simulink model "BrowarModel"  (R2024a)
settings: Solver=ode5  StartTime=0.0  StopTime=inf  FixedStep=0.1  RelTol=1e-3
undefined symbols (not defined in the file or in its folder): localhost, Matrikon, OI
libraries: opclib x24
(part 1 of 9)
settings Model: Creator=Administrator  LastModifiedBy=user
settings SolverCC: AlgebraicLoopSolver=TrustRegion
settings DataIOCC: LimitDataPoints=on  SaveFormat=Array  SignalLoggingSaveFormat=ModelDataLogs  ReturnWorkspaceOutputs=off
settings OptimizationCC: BlockReduction=off  BooleanDataType=off  BufferReuse=off  ExpressionDepthLimit=2147483647  InitFltsAndDblsToZero=on  LifeSpan=inf
settings DebuggingCC: UnderspecifiedInitializationDetection=Classic  MergeDetectMultiDrivingBlocksExec=none  SolverPrmCheckMsg=warning  FcnCallInpInsideContextMsg=warning  UnconnectedInputMsg=warning  UnconnectedOutputMsg=warning  UnconnectedLineMsg=warning  StateNameClashWarn=warning  SFUnexpectedBacktrackingDiag=warning  SFNoUnconditionalDefaultTransitionDiag=warning  SFExecutionAtInitializationDiag=none  ArithmeticOperatorsInVariantConditions=warning
settings HardwareCC: ProdBitPerPointer=32  ProdBitPerSizeT=32  ProdBitPerPtrDiffT=32  ProdLargestAtomicFloat=None  ProdIntDivRoundTo=Undefined  ProdEndianess=Unspecified  ProdWordSize=32  ProdHWDeviceType=32-bit Generic
settings ModelReferenceCC: EnableRefExpFcnMdlSchedulingChecks=on  PropagateSignalLabelsOutOfModel=off
settings SFSimCC: SimUseLocalCustomCode=off  CustomCodeUndefinedFunction=UseInterfaceOnly
settings RTWCC: RTWUseLocalCustomCode=off  GPUComputeCapability=3.5  DLArmComputeVersion=19.05
settings CodeAppCC: StateflowObjectComments=on
settings GRTTargetCC: TargetLangStandard=C89/C90 (ANSI)  CombineOutputUpdateFcns=off  GRTInterface=on
settings ConfigComp: CovMetricSettings=dw  CovSaveCumulativeToWorkspaceVar=on  CovSaveSingleToWorkspaceVar=on  CovExternalEMLEnable=off

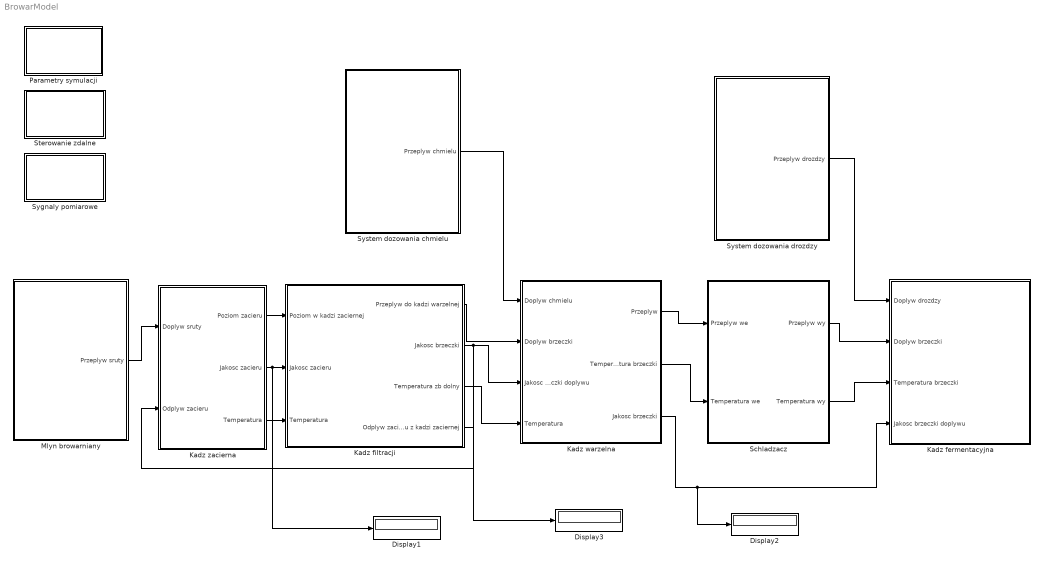
== system BrowarModel ==
  Display1 : Display
  Display2 : Display
  Display3 : Display
  Kadz fermentacyjna : Subsystem
  Kadz filtracji : Subsystem
  Kadz warzelna : Subsystem
  Kadz zacierna : Subsystem
  Mlyn browarniany : Subsystem
  Parametry symulacji : Subsystem
  Schladzacz : Subsystem
  Sterowanie zdalne : Subsystem
  Sygnaly pomiarowe : Subsystem
  System dozowania chmielu : Subsystem
  System dozowania drozdzy : Subsystem
  wires:
  Kadz filtracji/1(Przeplyw do kadzi warzelnej) -> Kadz warzelna/2(Doplyw brzeczki)
  System dozowania chmielu/1(Przeplyw chmielu) -> Kadz warzelna/1(Doplyw chmielu)
  Kadz warzelna/3(Jakosc brzeczki) -> Kadz fermentacyjna/4(Jakosc brzeczki doplywu), Display2/1
  Kadz filtracji/3(Temperatura zb dolny) -> Kadz warzelna/4(Temperatura)
  Kadz filtracji/2(Jakosc brzeczki) -> Kadz warzelna/3(Jakosc brzeczki doplywu), Display3/1
  Schladzacz/2(Temperatura wy) -> Kadz fermentacyjna/3(Temperatura brzeczki)
  Schladzacz/1(Przeplyw wy) -> Kadz fermentacyjna/2(Doplyw brzeczki)
  Kadz warzelna/1(Przeplyw) -> Schladzacz/1(Przeplyw we)
  Kadz warzelna/2(Temperatura brzeczki) -> Schladzacz/2(Temperatura we)
  System dozowania drozdzy/1(Przeplyw drozdzy) -> Kadz fermentacyjna/1(Doplyw drozdzy)
  Kadz filtracji/4(Odplyw zacieru z kadzi zaciernej) -> Kadz zacierna/2(Odplyw zacieru)
  Mlyn browarniany/1("Przeplyw sruty ") -> Kadz zacierna/1(Doplyw sruty)
  Kadz zacierna/1(Poziom zacieru) -> Kadz filtracji/1(Poziom w kadzi zaciernej)
  Kadz zacierna/2(Jakosc zacieru) -> Kadz filtracji/2(Jakosc zacieru), Display1/1
  Kadz zacierna/3(Temperatura) -> Kadz filtracji/3(Temperatura)

== system BrowarModel/Kadz fermentacyjna ==
  note: Kadz fermentacji
  Doplyw drozdzy : Inport
  Doplyw brzeczki : Inport  Port=2
  Temperatura brzeczki : Inport  Port=3
  Jakosc brzeczki doplywu : Inport  Port=4
  ET704 : Subsystem  mask{SrcZakres=12, Zakres=12, Kompensacja=0, ZakloceniaPom=off}
      mask prompts: SrcZakres "Zakres zmiennej w modelu"; Zakres "Zakres pomiarowy przetwornika pomiarowego"; Kompensacja "Kompensacja przetwornika pomiarowego"; ZakloceniaPom "Zaklocenia pomiarowe"
  ET705 : Subsystem  mask{SrcZakres=12, Zakres=12, Kompensacja=0, ZakloceniaPom=off}
      mask prompts: SrcZakres "Zakres zmiennej w modelu"; Zakres "Zakres pomiarowy przetwornika pomiarowego"; Kompensacja "Kompensacja przetwornika pomiarowego"; ZakloceniaPom "Zaklocenia pomiarowe"
  FV705 : Subsystem
  FV705SP : Subsystem
  FV706 : Subsystem
  Kadz fermentacyjna : Subsystem
  LT701 : Subsystem  mask{SrcZakres=3.5, Zakres=3.5, Kompensacja=0, ZakloceniaPom=on}
      mask prompts: SrcZakres "Zakres zmiennej w modelu"; Zakres "Zakres pomiarowy przetwornika pomiarowego"; Kompensacja "Kompensacja przetwornika pomiarowego"; ZakloceniaPom "Zaklocenia pomiarowe"
  LT701H : Subsystem
  LT701L : Subsystem
  ST704 : Subsystem  mask{SrcZakres=2000, Zakres=2000, Kompensacja=0, ZakloceniaPom=off}
      mask prompts: SrcZakres "Zakres zmiennej w modelu"; Zakres "Zakres pomiarowy przetwornika pomiarowego"; Kompensacja "Kompensacja przetwornika pomiarowego"; ZakloceniaPom "Zaklocenia pomiarowe"
  ST705 : Subsystem  mask{SrcZakres=2000, Zakres=2000, Kompensacja=0, ZakloceniaPom=off}
      mask prompts: SrcZakres "Zakres zmiennej w modelu"; Zakres "Zakres pomiarowy przetwornika pomiarowego"; Kompensacja "Kompensacja przetwornika pomiarowego"; ZakloceniaPom "Zaklocenia pomiarowe"
  TT702H : Subsystem  mask{SrcZakres=150, Zakres=150, Kompensacja=0, ZakloceniaPom=on}
      mask prompts: SrcZakres "Zakres zmiennej w modelu"; Zakres "Zakres pomiarowy przetwornika pomiarowego"; Kompensacja "Kompensacja przetwornika pomiarowego"; ZakloceniaPom "Zaklocenia pomiarowe"
  TT702L : Subsystem  mask{SrcZakres=150, Zakres=150, Kompensacja=0, ZakloceniaPom=on}
      mask prompts: SrcZakres "Zakres zmiennej w modelu"; Zakres "Zakres pomiarowy przetwornika pomiarowego"; Kompensacja "Kompensacja przetwornika pomiarowego"; ZakloceniaPom "Zaklocenia pomiarowe"
  TT702M : Subsystem  mask{SrcZakres=150, Zakres=150, Kompensacja=0, ZakloceniaPom=on}
      mask prompts: SrcZakres "Zakres zmiennej w modelu"; Zakres "Zakres pomiarowy przetwornika pomiarowego"; Kompensacja "Kompensacja przetwornika pomiarowego"; ZakloceniaPom "Zaklocenia pomiarowe"
  TV702 : Subsystem
  Terminator : Terminator
  XV704 : Subsystem
  XV704SP : Subsystem
  tag scope: ET704=global, ET705=global, LT701=global, LT701H=global, LT701L=global, Odplyw=global, ST704=global, ST705=global, TT702H=global, TT702L=global, TT702M=global, XV704Alarm=global, XV704Idle=global, XV704Running=global, XV705Alarm=global, XV705Idle=global, XV705Running=global
  wires:
  Kadz fermentacyjna/1(Poziom) -> LT701/1(In)
  Kadz fermentacyjna/2(Poziom wysoki) -> LT701H/1(In)
  Kadz fermentacyjna/3(Poziom niski) -> LT701L/1(In)
  Kadz fermentacyjna/5(Sensor temperatury gorny) -> TT702H/1(In)
  Kadz fermentacyjna/6(Sensor temperatury srodkowy) -> TT702M/1(In)
  Kadz fermentacyjna/7(Sensor temperatury dolny) -> TT702L/1(In)
  Kadz fermentacyjna/4(Temperatura) -> Terminator/1
  TV702/1(Out) -> Kadz fermentacyjna/3(Ster ogrzewaniem)
  XV704SP/1(Out) -> Kadz fermentacyjna/5("Zadane obroty silnika ")
  XV704/1(Out) -> Kadz fermentacyjna/4(Zalaczenie silnika)
  Kadz fermentacyjna/8(Obroty silnika) -> ST704/1(In)
  Kadz fermentacyjna/9(Prad silnika) -> ET704/1(In)
  Doplyw brzeczki/1 -> Kadz fermentacyjna/1(Doplyw brzeczki)
  Temperatura brzeczki/1 -> Kadz fermentacyjna/2(Temperatura brzeczki)
  LT701/1(Out) -> [LT701]
  LT701H/1(Out) -> [LT701H]
  LT701L/1(Out) -> [LT701L]
  TT702H/1(Out) -> [TT702H]
  TT702M/1(Out) -> [TT702M]
  TT702L/1(Out) -> [TT702L]
  ST704/1(Out) -> [ST704]
  ET704/1(Out) -> [ET704]
  Kadz fermentacyjna/10(Silnik Idle) -> [XV704Idle]
  Kadz fermentacyjna/11(Silnik Running) -> [XV704Running]
  Kadz fermentacyjna/12(Silnik Alarm) -> [XV704Alarm]
  ST705/1(Out) -> [ST705]
  ET705/1(Out) -> [ET705]
  Kadz fermentacyjna/15(Pompa odplywu Idle) -> [XV705Idle]
  Kadz fermentacyjna/16(Pompa odplywu Running) -> [XV705Running]
  Kadz fermentacyjna/17(Pompa odplywu Alarm) -> [XV705Alarm]
  Kadz fermentacyjna/13(Obroty pompy odplywu) -> ST705/1(In)
  Kadz fermentacyjna/14(Prad pompy odplywu) -> ET705/1(In)
  Kadz fermentacyjna/18(Przeplyw) -> [Odplyw]
  FV705/1(Out) -> Kadz fermentacyjna/7(Zalaczenie pompy)
  FV705SP/1(Out) -> Kadz fermentacyjna/8(Sterowanie pompy)
  FV706/1(Out) -> Kadz fermentacyjna/6(Sterowanie zaworem)
  Doplyw drozdzy/1 -> Kadz fermentacyjna/9(Doplyw drozdzy)
  Jakosc brzeczki doplywu/1 -> Kadz fermentacyjna/10(Jakosc brzeczki doplywu)

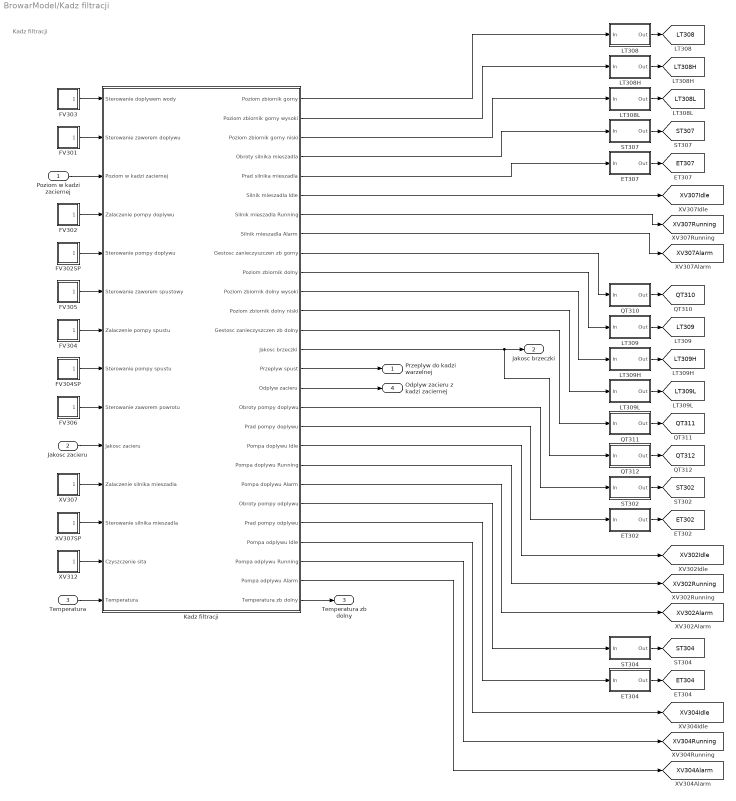
== system BrowarModel/Kadz filtracji ==
  note: Kadz filtracji
  Poziom w kadzi zaciernej : Inport
  Jakosc zacieru : Inport  Port=2
  Temperatura : Inport  Port=3
  ET302 : Subsystem  mask{SrcZakres=12, Zakres=12, Kompensacja=0, ZakloceniaPom=off}
      mask prompts: SrcZakres "Zakres zmiennej w modelu"; Zakres "Zakres pomiarowy przetwornika pomiarowego"; Kompensacja "Kompensacja przetwornika pomiarowego"; ZakloceniaPom "Zaklocenia pomiarowe"
  ET304 : Subsystem  mask{SrcZakres=12, Zakres=12, Kompensacja=0, ZakloceniaPom=off}
      mask prompts: SrcZakres "Zakres zmiennej w modelu"; Zakres "Zakres pomiarowy przetwornika pomiarowego"; Kompensacja "Kompensacja przetwornika pomiarowego"; ZakloceniaPom "Zaklocenia pomiarowe"
  ET307 : Subsystem  mask{SrcZakres=12, Zakres=12, Kompensacja=0, ZakloceniaPom=off}
      mask prompts: SrcZakres "Zakres zmiennej w modelu"; Zakres "Zakres pomiarowy przetwornika pomiarowego"; Kompensacja "Kompensacja przetwornika pomiarowego"; ZakloceniaPom "Zaklocenia pomiarowe"
  FV301 : Subsystem
  FV302 : Subsystem
  FV302SP : Subsystem
  FV303 : Subsystem
  FV304 : Subsystem
  FV304SP : Subsystem
  FV305 : Subsystem
  FV306 : Subsystem
  Kadz filtracji : Subsystem
  LT308 : Subsystem  mask{SrcZakres=2.5, Zakres=2.5, Kompensacja=0, ZakloceniaPom=on}
      mask prompts: SrcZakres "Zakres zmiennej w modelu"; Zakres "Zakres pomiarowy przetwornika pomiarowego"; Kompensacja "Kompensacja przetwornika pomiarowego"; ZakloceniaPom "Zaklocenia pomiarowe"
  LT308H : Subsystem
  LT308L : Subsystem
  LT309 : Subsystem  mask{SrcZakres=5, Zakres=5, Kompensacja=0, ZakloceniaPom=on}
      mask prompts: SrcZakres "Zakres zmiennej w modelu"; Zakres "Zakres pomiarowy przetwornika pomiarowego"; Kompensacja "Kompensacja przetwornika pomiarowego"; ZakloceniaPom "Zaklocenia pomiarowe"
  LT309H : Subsystem
  LT309L : Subsystem
  QT310 : Subsystem  mask{SrcZakres=1.1, Zakres=100, Kompensacja=0, ZakloceniaPom=on}
      mask prompts: SrcZakres "Zakres zmiennej w modelu"; Zakres "Zakres pomiarowy przetwornika pomiarowego"; Kompensacja "Kompensacja przetwornika pomiarowego"; ZakloceniaPom "Zaklocenia pomiarowe"
  QT311 : Subsystem  mask{SrcZakres=1.1, Zakres=100, Kompensacja=0, ZakloceniaPom=on}
      mask prompts: SrcZakres "Zakres zmiennej w modelu"; Zakres "Zakres pomiarowy przetwornika pomiarowego"; Kompensacja "Kompensacja przetwornika pomiarowego"; ZakloceniaPom "Zaklocenia pomiarowe"
  QT312 : Subsystem  mask{SrcZakres=100, Zakres=100, Kompensacja=0, ZakloceniaPom=on}
      mask prompts: SrcZakres "Zakres zmiennej w modelu"; Zakres "Zakres pomiarowy przetwornika pomiarowego"; Kompensacja "Kompensacja przetwornika pomiarowego"; ZakloceniaPom "Zaklocenia pomiarowe"
  ST302 : Subsystem  mask{SrcZakres=2000, Zakres=2000, Kompensacja=0, ZakloceniaPom=off}
      mask prompts: SrcZakres "Zakres zmiennej w modelu"; Zakres "Zakres pomiarowy przetwornika pomiarowego"; Kompensacja "Kompensacja przetwornika pomiarowego"; ZakloceniaPom "Zaklocenia pomiarowe"
  ST304 : Subsystem  mask{SrcZakres=2000, Zakres=2000, Kompensacja=0, ZakloceniaPom=off}
      mask prompts: SrcZakres "Zakres zmiennej w modelu"; Zakres "Zakres pomiarowy przetwornika pomiarowego"; Kompensacja "Kompensacja przetwornika pomiarowego"; ZakloceniaPom "Zaklocenia pomiarowe"
  ST307 : Subsystem  mask{SrcZakres=2000, Zakres=2000, Kompensacja=0, ZakloceniaPom=off}
      mask prompts: SrcZakres "Zakres zmiennej w modelu"; Zakres "Zakres pomiarowy przetwornika pomiarowego"; Kompensacja "Kompensacja przetwornika pomiarowego"; ZakloceniaPom "Zaklocenia pomiarowe"
  XV307 : Subsystem
  XV307SP : Subsystem
  XV312 : Subsystem
  Przeplyw do kadzi warzelnej : Outport
  Jakosc brzeczki : Outport  Port=2
  Temperatura zb dolny : Outport  Port=3
  Odplyw zacieru z kadzi zaciernej : Outport  Port=4
  tag scope: ET302=global, ET304=global, ET307=global, LT308=global, LT308H=global, LT308L=global, LT309=global, LT309H=global, LT309L=global, QT310=global, QT311=global, QT312=global, ST302=global, ST304=global, ST307=global, XV302Alarm=global, XV302Idle=global, XV302Running=global, XV304Alarm=global, XV304Idle=global, XV304Running=global, XV307Alarm=global, XV307Idle=global, XV307Running=global
  wires:
  FV303/1(Out) -> Kadz filtracji/1(Sterowanie doplywem wody)
  FV301/1(Out) -> Kadz filtracji/2(Sterowanie zaworem doplywu)
  FV302/1(Out) -> Kadz filtracji/4(Zalaczenie pompy doplywu)
  FV302SP/1(Out) -> Kadz filtracji/5(Sterowanie pompy doplywu)
  FV304/1(Out) -> Kadz filtracji/7(Zalaczenie pompy spustu)
  FV304SP/1(Out) -> Kadz filtracji/8(Sterowanie pompy spustu)
  FV305/1(Out) -> Kadz filtracji/6(Sterowanie zaworem spustowy)
  FV306/1(Out) -> Kadz filtracji/9(Sterowanie zaworem powrotu)
  XV307/1(Out) -> Kadz filtracji/11(Zalaczenie silnika mieszadla)
  XV307SP/1(Out) -> Kadz filtracji/12(Sterowanie silnika mieszadla)
  Kadz filtracji/1(Poziom zbiornik gorny) -> LT308/1(In)
  Kadz filtracji/9(Gestosc zanieczyszczen zb gorny) -> QT310/1(In)
  Kadz filtracji/14(Jakosc brzeczki) -> Jakosc brzeczki/1, QT312/1(In)
  Poziom w kadzi zaciernej/1 -> Kadz filtracji/3(Poziom w kadzi zaciernej)
  Jakosc zacieru/1 -> Kadz filtracji/10(Jakosc zacieru)
  Kadz filtracji/15(Przeplyw spust) -> Przeplyw do kadzi warzelnej/1
  LT308/1(Out) -> [LT308]
  LT308H/1(Out) -> [LT308H]
  Kadz filtracji/2(Poziom zbiornik gorny wysoki) -> LT308H/1(In)
  LT308L/1(Out) -> [LT308L]
  Kadz filtracji/3(Poziom zbiornik gorny niski) -> LT308L/1(In)
  ST307/1(Out) -> [ST307]
  ET307/1(Out) -> [ET307]
  Kadz filtracji/4(Obroty silnika mieszadla) -> ST307/1(In)
  Kadz filtracji/5(Prad silnika mieszadla) -> ET307/1(In)
  Kadz filtracji/6(Silnik mieszadla Idle) -> [XV307Idle]
  Kadz filtracji/7(Silnik mieszadla Running) -> [XV307Running]
  Kadz filtracji/8(Silnik mieszadla Alarm) -> [XV307Alarm]
  QT310/1(Out) -> [QT310]
  LT309/1(Out) -> [LT309]
  LT309H/1(Out) -> [LT309H]
  LT309L/1(Out) -> [LT309L]
  Kadz filtracji/10(Poziom zbiornik dolny) -> LT309/1(In)
  Kadz filtracji/11(Poziom zbiornik dolny wysoki) -> LT309H/1(In)
  Kadz filtracji/12(Poziom zbiornik dolny niski) -> LT309L/1(In)
  QT311/1(Out) -> [QT311]
  Kadz filtracji/13(Gestosc zanieczyszczen zb dolny) -> QT311/1(In)
  QT312/1(Out) -> [QT312]
  Kadz filtracji/16(Odplyw zacieru) -> Odplyw zacieru z kadzi zaciernej/1
  XV312/1(Out) -> Kadz filtracji/13(Czyszczenie sita)
  ET302/1(Out) -> [ET302]
  ST302/1(Out) -> [ST302]
  Kadz filtracji/17(Obroty pompy doplywu) -> ST302/1(In)
  Kadz filtracji/18(Prad pompy doplywu) -> ET302/1(In)
  Kadz filtracji/19(Pompa doplywu Idle) -> [XV302Idle]
  Kadz filtracji/20(Pompa doplywu Running) -> [XV302Running]
  Kadz filtracji/21(Pompa doplywu Alarm) -> [XV302Alarm]
  ET304/1(Out) -> [ET304]
  ST304/1(Out) -> [ST304]
  Kadz filtracji/22(Obroty pompy odplywu) -> ST304/1(In)
  Kadz filtracji/23(Prad pompy odplywu) -> ET304/1(In)
  Kadz filtracji/24(Pompa odplywu Idle) -> [XV304Idle]
  Kadz filtracji/25(Pompa odplywu Running) -> [XV304Running]
  Kadz filtracji/26(Pompa odplywu Alarm) -> [XV304Alarm]
  Temperatura/1 -> Kadz filtracji/14(Temperatura)
  Kadz filtracji/27(Temperatura zb dolny) -> Temperatura zb dolny/1

== system BrowarModel/Kadz warzelna ==
  note: Kadz warzelna
  Doplyw chmielu : Inport
  Doplyw brzeczki : Inport  Port=2
  Jakosc brzeczki doplywu : Inport  Port=3
  Temperatura : Inport  Port=4
  ET404 : Subsystem  mask{SrcZakres=12, Zakres=12, Kompensacja=0, ZakloceniaPom=off}
      mask prompts: SrcZakres "Zakres zmiennej w modelu"; Zakres "Zakres pomiarowy przetwornika pomiarowego"; Kompensacja "Kompensacja przetwornika pomiarowego"; ZakloceniaPom "Zaklocenia pomiarowe"
  FV404 : Subsystem
  FV404SP : Subsystem
  FV405 : Subsystem
  Kadz warzelna : Subsystem
  LT401 : Subsystem  mask{SrcZakres=3.5, Zakres=3.5, Kompensacja=0, ZakloceniaPom=on}
      mask prompts: SrcZakres "Zakres zmiennej w modelu"; Zakres "Zakres pomiarowy przetwornika pomiarowego"; Kompensacja "Kompensacja przetwornika pomiarowego"; ZakloceniaPom "Zaklocenia pomiarowe"
  LT401H : Subsystem
  LT401L : Subsystem
  ST404 : Subsystem  mask{SrcZakres=2000, Zakres=2000, Kompensacja=0, ZakloceniaPom=off}
      mask prompts: SrcZakres "Zakres zmiennej w modelu"; Zakres "Zakres pomiarowy przetwornika pomiarowego"; Kompensacja "Kompensacja przetwornika pomiarowego"; ZakloceniaPom "Zaklocenia pomiarowe"
  TT402H : Subsystem  mask{SrcZakres=150, Zakres=150, Kompensacja=0, ZakloceniaPom=on}
      mask prompts: SrcZakres "Zakres zmiennej w modelu"; Zakres "Zakres pomiarowy przetwornika pomiarowego"; Kompensacja "Kompensacja przetwornika pomiarowego"; ZakloceniaPom "Zaklocenia pomiarowe"
  TT402L : Subsystem  mask{SrcZakres=150, Zakres=150, Kompensacja=0, ZakloceniaPom=on}
      mask prompts: SrcZakres "Zakres zmiennej w modelu"; Zakres "Zakres pomiarowy przetwornika pomiarowego"; Kompensacja "Kompensacja przetwornika pomiarowego"; ZakloceniaPom "Zaklocenia pomiarowe"
  TT402M : Subsystem  mask{SrcZakres=150, Zakres=150, Kompensacja=0, ZakloceniaPom=on}
      mask prompts: SrcZakres "Zakres zmiennej w modelu"; Zakres "Zakres pomiarowy przetwornika pomiarowego"; Kompensacja "Kompensacja przetwornika pomiarowego"; ZakloceniaPom "Zaklocenia pomiarowe"
  TV402 : Subsystem
  Przeplyw : Outport
  Temperatura brzeczki : Outport  Port=2
  Jakosc brzeczki : Outport  Port=3
  tag scope: ET404=global, LT401=global, LT401H=global, LT401L=global, ST404=global, TT402H=global, TT402L=global, TT402M=global, XV404Alarm=global, XV404Idle=global, XV404Running=global
  wires:
  TV402/1(Out) -> Kadz warzelna/3(Ster ogrzew)
  Kadz warzelna/4(Temperatura) -> Temperatura brzeczki/1
  Doplyw chmielu/1 -> Kadz warzelna/1(Doplyw chmielu)
  Doplyw brzeczki/1 -> Kadz warzelna/2(Doplyw brzeczki)
  Jakosc brzeczki doplywu/1 -> Kadz warzelna/4(Jakosc brzeczki doplywu)
  LT401/1(Out) -> [LT401]
  LT401H/1(Out) -> [LT401H]
  LT401L/1(Out) -> [LT401L]
  Kadz warzelna/1(Poziom) -> LT401/1(In)
  Kadz warzelna/2(Poziom wysoki) -> LT401H/1(In)
  Kadz warzelna/3(Poziom niski) -> LT401L/1(In)
  TT402H/1(Out) -> [TT402H]
  TT402M/1(Out) -> [TT402M]
  TT402L/1(Out) -> [TT402L]
  Kadz warzelna/5(Sensor temperatury gorny) -> TT402H/1(In)
  Kadz warzelna/6(Sensor temperatury srodkowy) -> TT402M/1(In)
  Kadz warzelna/7(Sensor temperatury dolny) -> TT402L/1(In)
  Kadz warzelna/8(Jakosc brzeczki) -> Jakosc brzeczki/1
  Kadz warzelna/14(Przeplyw) -> Przeplyw/1
  ET404/1(Out) -> [ET404]
  ST404/1(Out) -> [ST404]
  Kadz warzelna/9(Obroty pompy odplywu) -> ST404/1(In)
  Kadz warzelna/10(Prad pompy odplywu) -> ET404/1(In)
  Kadz warzelna/11(Pompa odplywu Idle) -> [XV404Idle]
  Kadz warzelna/12(Pompa odplywu Running) -> [XV404Running]
  Kadz warzelna/13(Pompa odplywu Alarm) -> [XV404Alarm]
  FV405/1(Out) -> Kadz warzelna/5(Sterowanie zaworem)
  FV404/1(Out) -> Kadz warzelna/6(Zalaczenie pompy)
  FV404SP/1(Out) -> Kadz warzelna/7(Sterowanie pompy)
  Temperatura/1 -> Kadz warzelna/8(Temp doplywu)

== system BrowarModel/Kadz zacierna ==
  note: Kadz zacierna
  Doplyw sruty : Inport
  Odplyw zacieru : Inport  Port=2
  ET205 : Subsystem  mask{SrcZakres=12, Zakres=12, Kompensacja=0, ZakloceniaPom=off}
      mask prompts: SrcZakres "Zakres zmiennej w modelu"; Zakres "Zakres pomiarowy przetwornika pomiarowego"; Kompensacja "Kompensacja przetwornika pomiarowego"; ZakloceniaPom "Zaklocenia pomiarowe"
  FT201 : Subsystem  mask{SrcZakres=0.25, Zakres=250, Kompensacja=0, ZakloceniaPom=on}
      mask prompts: SrcZakres "Zakres zmiennej w modelu"; Zakres "Zakres pomiarowy przetwornika pomiarowego"; Kompensacja "Kompensacja przetwornika pomiarowego"; ZakloceniaPom "Zaklocenia pomiarowe"
  Kadz zacierna : Subsystem
  LT202 : Subsystem  mask{SrcZakres=2, Zakres=2, Kompensacja=0, ZakloceniaPom=on}
      mask prompts: SrcZakres "Zakres zmiennej w modelu"; Zakres "Zakres pomiarowy przetwornika pomiarowego"; Kompensacja "Kompensacja przetwornika pomiarowego"; ZakloceniaPom "Zaklocenia pomiarowe"
  LT202H : Subsystem
  LT202L : Subsystem
  LV201 : Subsystem
  QT204 : Subsystem
  ST205 : Subsystem  mask{SrcZakres=2000, Zakres=2000, Kompensacja=0, ZakloceniaPom=off}
      mask prompts: SrcZakres "Zakres zmiennej w modelu"; Zakres "Zakres pomiarowy przetwornika pomiarowego"; Kompensacja "Kompensacja przetwornika pomiarowego"; ZakloceniaPom "Zaklocenia pomiarowe"
  TT203H : Subsystem  mask{SrcZakres=150, Zakres=150, Kompensacja=0, ZakloceniaPom=on}
      mask prompts: SrcZakres "Zakres zmiennej w modelu"; Zakres "Zakres pomiarowy przetwornika pomiarowego"; Kompensacja "Kompensacja przetwornika pomiarowego"; ZakloceniaPom "Zaklocenia pomiarowe"
  TT203L : Subsystem  mask{SrcZakres=150, Zakres=150, Kompensacja=0, ZakloceniaPom=on}
      mask prompts: SrcZakres "Zakres zmiennej w modelu"; Zakres "Zakres pomiarowy przetwornika pomiarowego"; Kompensacja "Kompensacja przetwornika pomiarowego"; ZakloceniaPom "Zaklocenia pomiarowe"
  TT203M : Subsystem  mask{SrcZakres=150, Zakres=150, Kompensacja=0, ZakloceniaPom=on}
      mask prompts: SrcZakres "Zakres zmiennej w modelu"; Zakres "Zakres pomiarowy przetwornika pomiarowego"; Kompensacja "Kompensacja przetwornika pomiarowego"; ZakloceniaPom "Zaklocenia pomiarowe"
  TV203 : Subsystem
  XV205 : Subsystem
  XV205SP : Subsystem
  Poziom zacieru : Outport
  Jakosc zacieru : Outport  Port=2
  Temperatura : Outport  Port=3
  tag scope: ET205=global, FT201=global, LT202=global, LT202H=global, LT202L=global, QT204=global, ST205=global, TT203H=global, TT203L=global, TT203M=global, XV205Alarm=global, XV205Idle=global, XV205Running=global
  wires:
  LV201/1(Out) -> Kadz zacierna/1("Doplyw wody ")
  Kadz zacierna/1(Poziom) -> Poziom zacieru/1, LT202/1(In)
  XV205/1(Out) -> Kadz zacierna/3(Zalaczenie silnika)
  XV205SP/1(Out) -> Kadz zacierna/4("Zadane obroty silnika ")
  TV203/1(Out) -> Kadz zacierna/5(Sterowanie ogrzewaczem)
  LT202H/1(Out) -> [LT202H]
  FT201/1(Out) -> [FT201]
  Kadz zacierna/4(Przeplyw wody) -> FT201/1(In)
  Kadz zacierna/2(Poziom wysoki) -> LT202H/1(In)
  LT202/1(Out) -> [LT202]
  LT202L/1(Out) -> [LT202L]
  Kadz zacierna/3(Poziom niski) -> LT202L/1(In)
  Doplyw sruty/1 -> Kadz zacierna/2(Doplyw sruty)
  Odplyw zacieru/1 -> Kadz zacierna/6(Odplyw)
  TT203H/1(Out) -> [TT203H]
  TT203M/1(Out) -> [TT203M]
  TT203L/1(Out) -> [TT203L]
  Kadz zacierna/5(Sensor temperatury gorny) -> TT203H/1(In)
  Kadz zacierna/6(Sensor temperatury srodkowy) -> TT203M/1(In)
  Kadz zacierna/7(Sensor temperatury dolny) -> TT203L/1(In)
  ST205/1(Out) -> [ST205]
  ET205/1(Out) -> [ET205]
  Kadz zacierna/8(Obroty silnika) -> ST205/1(In)
  Kadz zacierna/9(Prad silnika) -> ET205/1(In)
  QT204/1(Out) -> [QT204]
  Kadz zacierna/13(Jakosc zacieru) -> Jakosc zacieru/1, QT204/1(In)
  Kadz zacierna/10(Silnik Idle) -> [XV205Idle]
  Kadz zacierna/11(Silnik Running) -> [XV205Running]
  Kadz zacierna/12(Silnik Alarm) -> [XV205Alarm]
  Kadz zacierna/14(Temperatura) -> Temperatura/1

== system BrowarModel/Mlyn browarniany ==
  note: Mlyn browarniany
  ET103 : Subsystem  mask{SrcZakres=12, Zakres=12, Kompensacja=0, ZakloceniaPom=off}
      mask prompts: SrcZakres "Zakres zmiennej w modelu"; Zakres "Zakres pomiarowy przetwornika pomiarowego"; Kompensacja "Kompensacja przetwornika pomiarowego"; ZakloceniaPom "Zaklocenia pomiarowe"
  ET105 : Subsystem  mask{SrcZakres=12, Zakres=12, Kompensacja=0, ZakloceniaPom=off}
      mask prompts: SrcZakres "Zakres zmiennej w modelu"; Zakres "Zakres pomiarowy przetwornika pomiarowego"; Kompensacja "Kompensacja przetwornika pomiarowego"; ZakloceniaPom "Zaklocenia pomiarowe"
  FT105 : Subsystem  mask{SrcZakres=0.2, Zakres=200, Kompensacja=0, ZakloceniaPom=on}
      mask prompts: SrcZakres "Zakres zmiennej w modelu"; Zakres "Zakres pomiarowy przetwornika pomiarowego"; Kompensacja "Kompensacja przetwornika pomiarowego"; ZakloceniaPom "Zaklocenia pomiarowe"
  FV103 : Subsystem
  FV103SP : Subsystem
  FV105 : Subsystem
  FV105SP : Subsystem
  LT102 : Subsystem  mask{SrcZakres=6, Zakres=6, Kompensacja=0, ZakloceniaPom=on}
      mask prompts: SrcZakres "Zakres zmiennej w modelu"; Zakres "Zakres pomiarowy przetwornika pomiarowego"; Kompensacja "Kompensacja przetwornika pomiarowego"; ZakloceniaPom "Zaklocenia pomiarowe"
  LT102H : Subsystem
  LT102L : Subsystem
  LT104H : Subsystem
  LT104L : Subsystem
  LV101 : Subsystem
  Mlyn browarniany : Subsystem
  ST103 : Subsystem  mask{SrcZakres=2000, Zakres=2000, Kompensacja=0, ZakloceniaPom=off}
      mask prompts: SrcZakres "Zakres zmiennej w modelu"; Zakres "Zakres pomiarowy przetwornika pomiarowego"; Kompensacja "Kompensacja przetwornika pomiarowego"; ZakloceniaPom "Zaklocenia pomiarowe"
  ST105 : Subsystem  mask{SrcZakres=2000, Zakres=2000, Kompensacja=0, ZakloceniaPom=off}
      mask prompts: SrcZakres "Zakres zmiennej w modelu"; Zakres "Zakres pomiarowy przetwornika pomiarowego"; Kompensacja "Kompensacja przetwornika pomiarowego"; ZakloceniaPom "Zaklocenia pomiarowe"
  TT103 : Subsystem  mask{SrcZakres=300, Zakres=300, Kompensacja=0, ZakloceniaPom=on}
      mask prompts: SrcZakres "Zakres zmiennej w modelu"; Zakres "Zakres pomiarowy przetwornika pomiarowego"; Kompensacja "Kompensacja przetwornika pomiarowego"; ZakloceniaPom "Zaklocenia pomiarowe"
  TT105 : Subsystem  mask{SrcZakres=300, Zakres=300, Kompensacja=0, ZakloceniaPom=on}
      mask prompts: SrcZakres "Zakres zmiennej w modelu"; Zakres "Zakres pomiarowy przetwornika pomiarowego"; Kompensacja "Kompensacja przetwornika pomiarowego"; ZakloceniaPom "Zaklocenia pomiarowe"
  "Przeplyw sruty " : Outport
  tag scope: ET103=global, ET105=global, FT105=global, FV103Alarm=global, FV103Idle=global, FV103Running=global, FV105Alarm=global, FV105Running=global, FV105dle=global, LT102=global, LT102H=global, LT102L=global, LT104H=global, LT104L=global, ST103=global, ST105=global, TT103=global, TT105=global
  wires:
  LV101/1(Out) -> Mlyn browarniany/1(Doplyw zasobnika)
  FV103/1(Out) -> Mlyn browarniany/2(Zalaczenie silnika dozownika)
  FV103SP/1(Out) -> Mlyn browarniany/3(Zadane obroty silnika dozownika)
  FV105SP/1(Out) -> Mlyn browarniany/5(Zadane obroty silnika walcow)
  FV105/1(Out) -> Mlyn browarniany/4(Zalaczenie silnika walcow)
  LT102H/1(Out) -> [LT102H]
  Mlyn browarniany/1(Przeplyw) -> "Przeplyw sruty "/1, FT105/1(In)
  LT102/1(Out) -> [LT102]
  Mlyn browarniany/2(Poziom zasobnika) -> LT102/1(In)
  LT102L/1(Out) -> [LT102L]
  Mlyn browarniany/4(Poziom niski zasobnika) -> LT102L/1(In)
  Mlyn browarniany/3(Poziom wysoki zasobnika) -> LT102H/1(In)
  FT105/1(Out) -> [FT105]
  Mlyn browarniany/10(Temperatura lozyska dozownika) -> TT103/1(In)
  TT103/1(Out) -> [TT103]
  ST103/1(Out) -> [ST103]
  Mlyn browarniany/5(Obroty silnika dozownika) -> ST103/1(In)
  ET103/1(Out) -> [ET103]
  Mlyn browarniany/6(Prad silnika dozownika) -> ET103/1(In)
  Mlyn browarniany/7(Silnik dozownika Idle) -> [FV103Idle]
  Mlyn browarniany/8(Silnik dozownika Running) -> [FV103Running]
  Mlyn browarniany/9(Silnik dozownika Alarm) -> [FV103Alarm]
  LT104H/1(Out) -> [LT104H]
  LT104L/1(Out) -> [LT104L]
  Mlyn browarniany/11(Poziom wysoki komory) -> LT104H/1(In)
  Mlyn browarniany/12(Poziom niski komory) -> LT104L/1(In)
  ST105/1(Out) -> [ST105]
  ET105/1(Out) -> [ET105]
  Mlyn browarniany/15(Silnik walcow Idle) -> [FV105dle]
  Mlyn browarniany/16(Silnik walcow Running) -> [FV105Running]
  Mlyn browarniany/17(Silnik walcow Alarm) -> [FV105Alarm]
  TT105/1(Out) -> [TT105]
  Mlyn browarniany/18(Temperatura lozyska walcow) -> TT105/1(In)
  Mlyn browarniany/13(Obroty silnika walcow) -> ST105/1(In)
  Mlyn browarniany/14(Prad silnika walcow) -> ET105/1(In)

== system BrowarModel/Parametry symulacji ==
  note: Parametry symulacji
  Display : Display
  Display1 : Display
  OPC Configuration : opclib/OPC Configuration  opcServers=localhost/Matrikon.OPC.Simulation.1/10, localhost/OI.GATEWAY.3/10  errMissingItems=Error  errReadWrite=Warn  errShutdown=Error  errRTViolation=Warn  rtEnable=on  speedup=1  showLatency=on  beingUsed=on
  SimulinkVer : Constant  Value=0.91
  Terminator : Terminator
  TrybSter : Constant
  TrybSym : Constant
  ZaklPom : Constant
  ZaklProc : Constant
  Zegar : Clock
  tag scope: TrybSter=global, TrybSym=global, ZaklPom=global, ZaklProc=global
  wires:
  Zegar/1 -> Display/1
  TrybSter/1 -> [TrybSter]
  ZaklPom/1 -> [ZaklPom]
  ZaklProc/1 -> [ZaklProc]
  SimulinkVer/1 -> Terminator/1
  TrybSym/1 -> [TrybSym]
  OPC Configuration/1 -> Display1/1

== system BrowarModel/Schladzacz ==
  note: Schladzacz
  Przeplyw we : Inport
  Temperatura we : Inport  Port=2
  Schladzacz : Subsystem
  TT601 : Subsystem  mask{SrcZakres=150, Zakres=150, Kompensacja=0, ZakloceniaPom=on}
      mask prompts: SrcZakres "Zakres zmiennej w modelu"; Zakres "Zakres pomiarowy przetwornika pomiarowego"; Kompensacja "Kompensacja przetwornika pomiarowego"; ZakloceniaPom "Zaklocenia pomiarowe"
  TT602 : Subsystem  mask{SrcZakres=150, Zakres=150, Kompensacja=0, ZakloceniaPom=on}
      mask prompts: SrcZakres "Zakres zmiennej w modelu"; Zakres "Zakres pomiarowy przetwornika pomiarowego"; Kompensacja "Kompensacja przetwornika pomiarowego"; ZakloceniaPom "Zaklocenia pomiarowe"
  TT603 : Subsystem  mask{SrcZakres=150, Zakres=150, Kompensacja=0, ZakloceniaPom=on}
      mask prompts: SrcZakres "Zakres zmiennej w modelu"; Zakres "Zakres pomiarowy przetwornika pomiarowego"; Kompensacja "Kompensacja przetwornika pomiarowego"; ZakloceniaPom "Zaklocenia pomiarowe"
  TT604 : Subsystem  mask{SrcZakres=150, Zakres=150, Kompensacja=0, ZakloceniaPom=on}
      mask prompts: SrcZakres "Zakres zmiennej w modelu"; Zakres "Zakres pomiarowy przetwornika pomiarowego"; Kompensacja "Kompensacja przetwornika pomiarowego"; ZakloceniaPom "Zaklocenia pomiarowe"
  TV601 : Subsystem
  Przeplyw wy : Outport
  Temperatura wy : Outport  Port=2
  tag scope: TT601=global, TT602=global, TT603=global, TT604=global
  wires:
  TT601/1(Out) -> [TT601]
  TT602/1(Out) -> [TT602]
  TT603/1(Out) -> [TT603]
  TT604/1(Out) -> [TT604]
  Temperatura we/1 -> Schladzacz/1(Temperatura we), TT602/1(In)
  Schladzacz/1(Temperatura wy) -> Temperatura wy/1, TT604/1(In)
  Przeplyw we/1 -> Schladzacz/2(Przeplyw we)
  Schladzacz/2(Przeplyw wy) -> Przeplyw wy/1
  TV601/1(Out) -> Schladzacz/3(Sterowanie)
  Schladzacz/3(Temperatura wody we) -> TT601/1(In)
  Schladzacz/4(Temperatura wody wy) -> TT603/1(In)

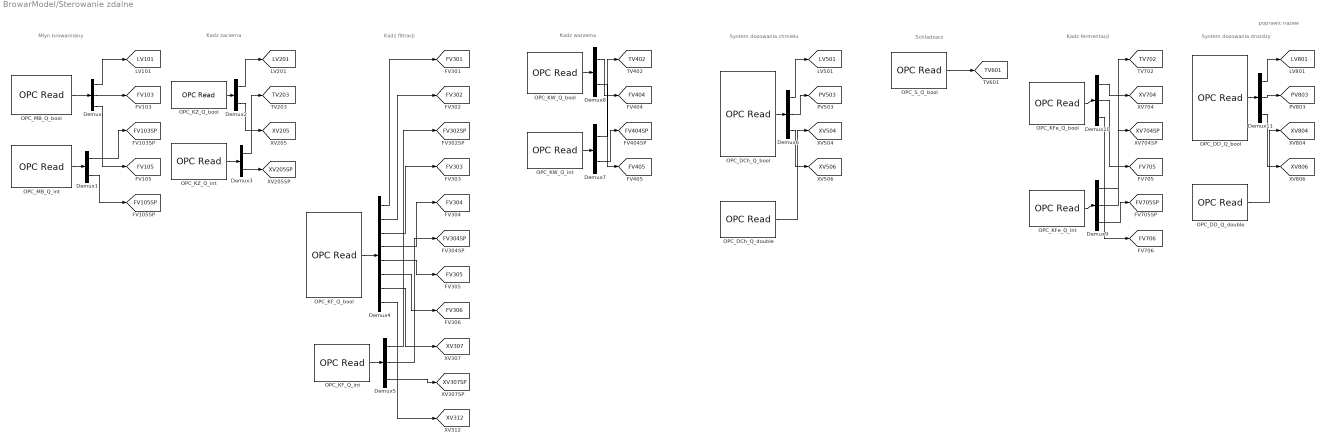
== system BrowarModel/Sterowanie zdalne ==
  note: Mlyn browarniany
  note: Kadz zacierna
  note: Kadz filtracji
  note: Kadz warzelna
  note: System dozowania chmielu
  note: Schladzacz
  note: Kadz fermentacji
  note: System dozowania drozdzy
  note: poprawic nazwe
  Demux{,5..6,9..11} (6 alike) : Demux  Outputs=3
  Demux{1..3,7..8} (5 alike) : Demux  Outputs=2
  Demux4 : Demux  Outputs=8
  OPC_DCh_Q_bool : opclib/OPC Read  serverHost=localhost  serverID=OI.GATEWAY.3  itemIDs=Bucket Brigade.DCh_Q_LV501, Bucket Brigade.DCh_Q_PV503, Bucket Brigade.DCh_Q_XV506  readMode=Synchronous (cache)  dataType=logical  updateRate=0.5  showQual=off  showTS=off  tsMode=Seconds since start
  OPC_DCh_Q_double : opclib/OPC Read  serverHost=localhost  serverID=OI.GATEWAY.3  itemIDs=Bucket Brigade.DCh_Q_XV504  readMode=Synchronous (cache)  dataType=double  updateRate=0.5  showQual=off  showTS=off  tsMode=Seconds since start
  OPC_DD_Q_bool : opclib/OPC Read  serverHost=localhost  serverID=OI.GATEWAY.3  itemIDs=Bucket Brigade.DD_Q_LV801, Bucket Brigade.DD_Q_PV803, Bucket Brigade.DD_Q_XV806  readMode=Synchronous (cache)  dataType=logical  updateRate=0.5  showQual=off  showTS=off  tsMode=Seconds since start
  OPC_DD_Q_double : opclib/OPC Read  serverHost=localhost  serverID=OI.GATEWAY.3  itemIDs=Bucket Brigade.DD_Q_XV804  readMode=Synchronous (cache)  dataType=double  updateRate=0.5  showQual=off  showTS=off  tsMode=Seconds since start
  OPC_KF_Q_bool : opclib/OPC Read  serverHost=localhost  serverID=OI.GATEWAY.3  itemIDs=Bucket Brigade.KF_Q_FV301, Bucket Brigade.KF_Q_FV302, Bucket Brigade.KF_Q_FV303, Bucket Brigade.KF_Q_FV304, Bucket Brigade.KF_Q_FV305, Bucket Brigade.KF_Q_FV306, Bucket Brigade.KF_Q_XV307, Bucket Brigade.KF_Q_XV312  readMode=Synchronous (cache)  dataType=logical  updateRate=0.5  showQual=off  showTS=off  tsMode=Seconds since start
  OPC_KF_Q_int : opclib/OPC Read  serverHost=localhost  serverID=OI.GATEWAY.3  itemIDs=Bucket Brigade.KF_Q_FV302SP, Bucket Brigade.KF_Q_FV304SP, Bucket Brigade.KF_Q_XV307SP  readMode=Synchronous (cache)  dataType=int16  updateRate=0.5  showQual=off  showTS=off  tsMode=Seconds since start
  OPC_KFe_Q_bool : opclib/OPC Read  serverHost=localhost  serverID=OI.GATEWAY.3  itemIDs=Bucket Brigade.KFe_Q_XV704, Bucket Brigade.KFe_Q_FV705, Bucket Brigade.KFe_Q_FV706  readMode=Synchronous (cache)  dataType=logical  updateRate=0.5  showQual=off  showTS=off  tsMode=Seconds since start
  OPC_KFe_Q_int : opclib/OPC Read  serverHost=localhost  serverID=OI.GATEWAY.3  itemIDs=Bucket Brigade.KFe_Q_TV702, Bucket Brigade.KFe_Q_XV704SP, Bucket Brigade.KFe_Q_FV705SP  readMode=Synchronous (cache)  dataType=int16  updateRate=0.5  showQual=off  showTS=off  tsMode=Seconds since start
  OPC_KW_Q_bool : opclib/OPC Read  serverHost=localhost  serverID=OI.GATEWAY.3  itemIDs=Bucket Brigade.KW_Q_FV404, Bucket Brigade.KW_Q_FV405  readMode=Synchronous (cache)  dataType=logical  updateRate=0.5  showQual=off  showTS=off  tsMode=Seconds since start
  OPC_KW_Q_int : opclib/OPC Read  serverHost=localhost  serverID=OI.GATEWAY.3  itemIDs=Bucket Brigade.KW_Q_TV402, Bucket Brigade.KW_Q_FV404SP  readMode=Synchronous (cache)  dataType=int16  updateRate=0.5  showQual=off  showTS=off  tsMode=Seconds since start
  OPC_KZ_Q_bool : opclib/OPC Read  serverHost=localhost  serverID=OI.GATEWAY.3  itemIDs=Bucket Brigade.KZ_Q_LV201, Bucket Brigade.KZ_Q_XV205  readMode=Synchronous (cache)  dataType=logical  updateRate=0.5  showQual=off  showTS=off  tsMode=Seconds since start
  OPC_KZ_Q_int : opclib/OPC Read  serverHost=localhost  serverID=OI.GATEWAY.3  itemIDs=Bucket Brigade.KZ_Q_TV203, Bucket Brigade.KZ_Q_XV205SP  readMode=Synchronous (cache)  dataType=int16  updateRate=0.5  showQual=off  showTS=off  tsMode=Seconds since start
  OPC_MB_Q_bool : opclib/OPC Read  serverHost=localhost  serverID=OI.GATEWAY.3  itemIDs=Bucket Brigade.MB_Q_LV101, Bucket Brigade.MB_Q_FV103, Bucket Brigade.MB_Q_FV105  readMode=Synchronous (cache)  dataType=logical  updateRate=0.5  showQual=off  showTS=off  tsMode=Seconds since start
  OPC_MB_Q_int : opclib/OPC Read  serverHost=localhost  serverID=OI.GATEWAY.3  itemIDs=Bucket Brigade.MB_Q_FV103SP, Bucket Brigade.MB_Q_FV105SP  readMode=Synchronous (cache)  dataType=int16  updateRate=0.5  showQual=off  showTS=off  tsMode=Seconds since start
  OPC_S_Q_bool : opclib/OPC Read  serverHost=localhost  serverID=OI.GATEWAY.3  itemIDs=Bucket Brigade.S_Q_TV601  readMode=Synchronous (cache)  dataType=logical  updateRate=0.5  showQual=off  showTS=off  tsMode=Seconds since start
  tag scope: FV103=global, FV103SP=global, FV105=global, FV105SP=global, FV301=global, FV302=global, FV302SP=global, FV303=global, FV304=global, FV304SP=global, FV305=global, FV306=global, FV404=global, FV404SP=global, FV405=global, FV705=global, FV705SP=global, FV706=global, LV101=global, LV201=global, LV501=global, LV801=global, PV503=global, PV803=global, TV203=global, TV402=global, TV601=global, TV702=global, XV205=global, XV205SP=global, XV307=global, XV307SP=global, XV312=global, XV504=global, XV506=global, XV704=global, XV704SP=global, XV804=global, XV806=global
  wires:
  OPC_MB_Q_bool/1 -> Demux/1
  Demux/1 -> [LV101]
  Demux/2 -> [FV103]
  Demux/3 -> [FV105]
  OPC_MB_Q_int/1 -> Demux1/1
  Demux1/1 -> [FV103SP]
  Demux1/2 -> [FV105SP]
  OPC_KZ_Q_int/1 -> Demux3/1
  OPC_KZ_Q_bool/1 -> Demux2/1
  Demux2/1 -> [LV201]
  Demux2/2 -> [XV205]
  Demux3/1 -> [TV203]
  Demux3/2 -> [XV205SP]
  OPC_KF_Q_bool/1 -> Demux4/1
  Demux4/1 -> [FV301]
  Demux4/2 -> [FV302]
  Demux4/3 -> [FV303]
  Demux4/4 -> [FV304]
  Demux4/5 -> [FV305]
  Demux4/6 -> [FV306]
  Demux4/7 -> [XV307]
  Demux4/8 -> [XV312]
  OPC_KF_Q_int/1 -> Demux5/1
  Demux5/1 -> [FV302SP]
  Demux5/2 -> [FV304SP]
  Demux5/3 -> [XV307SP]
  OPC_DCh_Q_bool/1 -> Demux6/1
  Demux6/1 -> [LV501]
  Demux6/2 -> [PV503]
  Demux6/3 -> [XV506]
  OPC_DCh_Q_double/1 -> [XV504]
  OPC_S_Q_bool/1 -> [TV601]
  OPC_KW_Q_int/1 -> Demux7/1
  OPC_KW_Q_bool/1 -> Demux8/1
  Demux8/1 -> [FV404]
  Demux8/2 -> [FV405]
  Demux7/1 -> [TV402]
  Demux7/2 -> [FV404SP]
  OPC_KFe_Q_int/1 -> Demux9/1
  OPC_KFe_Q_bool/1 -> Demux10/1
  Demux10/1 -> [XV704]
  Demux10/2 -> [FV705]
  Demux10/3 -> [FV706]
  Demux9/1 -> [TV702]
  Demux9/2 -> [XV704SP]
  Demux9/3 -> [FV705SP]
  OPC_DD_Q_bool/1 -> Demux11/1
  Demux11/1 -> [LV801]
  Demux11/2 -> [PV803]
  Demux11/3 -> [XV806]
  OPC_DD_Q_double/1 -> [XV804]

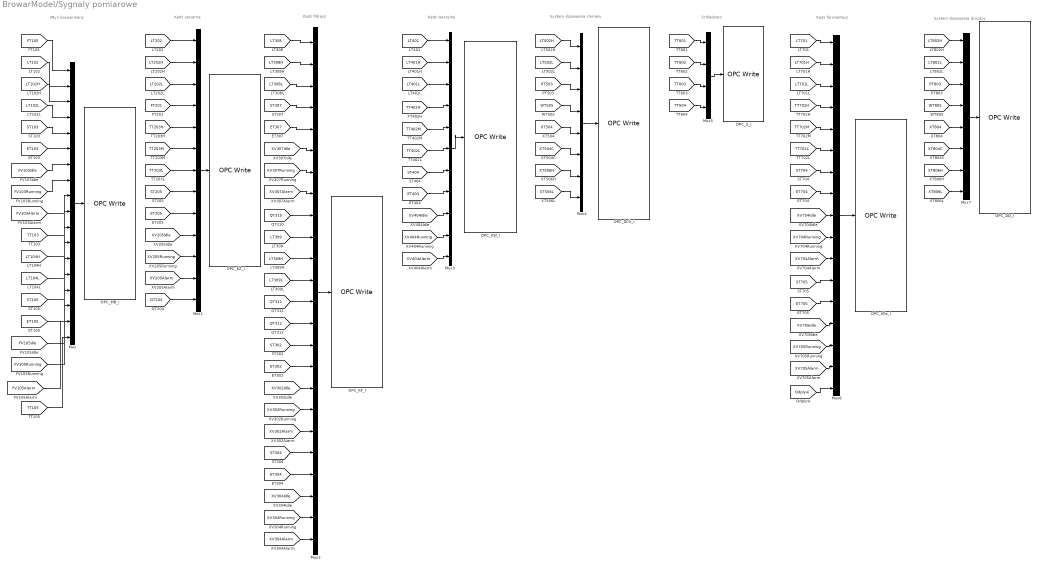
== system BrowarModel/Sygnaly pomiarowe ==
  note: Mlyn browarniany
  note: Kadz zacierna
  note: Kadz filtracji
  note: Kadz warzelna
  note: System dozowania chmielu
  note: Schladzacz
  note: Kadz fermentacji
  note: System dozowania drozdzy
  Mux : Mux  Inputs=18
  Mux1 : Mux  Inputs=13
  Mux2 : Mux  Inputs=24
  Mux3 : Mux  Inputs=11
  Mux4 : Mux  Inputs=8
  Mux5 : Mux
  Mux6 : Mux  Inputs=17
  Mux7 : Mux  Inputs=8
  OPC_DCh_I : opclib/OPC Write  serverHost=localhost  serverID=OI.GATEWAY.3  itemIDs=Bucket Brigade.DCh_I_LT502H, Bucket Brigade.DCh_I_LT502L, Bucket Brigade.DCh_I_PT503, Bucket Brigade.DCh_I_WT505, Bucket Brigade.DCh_I_XT504, Bucket Brigade.DCh_I_XT504C, Bucket Brigade.DCh_I_XT506H, Bucket Brigade.DCh_I_XT506L  writeMode=Synchronous  updateRate=1
  OPC_DD_I : opclib/OPC Write  serverHost=localhost  serverID=Matrikon.OPC.Simulation.1  itemIDs=Bucket Brigade.DD_I_LT802H, Bucket Brigade.KFe_I_LT802L, Bucket Brigade.KFe_I_PT803, Bucket Brigade.KFe_I_WT805, Bucket Brigade.KFe_I_XT804, Bucket Brigade.KFe_I_XT804C, Bucket Brigade.KFe_I_XT806H, Bucket Brigade.KFe_I_XT806L  writeMode=Synchronous  updateRate=1
  OPC_KF_I : opclib/OPC Write  serverHost=localhost  serverID=OI.GATEWAY.3  itemIDs=Bucket Brigade.KF_I_LT308, Bucket Brigade.KF_I_LT308H, Bucket Brigade.KF_I_LT308L, Bucket Brigade.KF_I_ST307, Bucket Brigade.KF_I_ET307, Bucket Brigade.KF_I_XV307Idle, Bucket Brigade.KF_I_XV307Running, Bucket Brigade.KF_I_XV307Alarm, Bucket Brigade.KF_I_QT310, Bucket Brigade.KF_I_LT309, Bucket Brigade.KF_I_LT309H, Bucket Brigade.KF_I_LT309L, Bucket Brigade.KF_I_QT311, Bucket Brigade.KF_I_QT312, Bucket Brigade.KF_I_ST302, Bucket Brigade.KF_I_ET302, Bucket Brigade.KF_I_XV302Idle, Bucket Brigade.KF_I_XC302Running, Bucket Brigade.KF_I_XV302Alarm, Bucket Brigade.KF_I_ST304, Bucket Brigade.KF_I_ET304, Bucket Brigade.KF_I_XV304Idle, Bucket Brigade.KF_I_XV304Running, Bucket Brigade.KF_I_XV304Alarm  writeMode=Synchronous  updateRate=1
  OPC_KFe_I : opclib/OPC Write  serverHost=localhost  serverID=Matrikon.OPC.Simulation.1  itemIDs=Bucket Brigade.KFe_I_LT701, Bucket Brigade.KFe_I_LT701H, Bucket Brigade.KFe_I_LT701L, Bucket Brigade.KFe_I_TT702H, Bucket Brigade.KFe_I_TT702M, Bucket Brigade.KFe_I_TT702L, Bucket Brigade.KFe_I_ST704, Bucket Brigade.KFe_I_ET704, Bucket Brigade.KFe_I_XV704Idle, Bucket Brigade.KFe_I_XV704Running, Bucket Brigade.KFe_I_XV704Alarm, Bucket Brigade.KFe_I_ST705, Bucket Brigade.KFe_I_ET705, Bucket Brigade.KFe_I_XV705Idle, Bucket Brigade.KFe_I_XV705Running, Bucket Brigade.KFe_I_XV705Alarm, Bucket Brigade.KFe_I_Odplyw  writeMode=Synchronous  updateRate=1
  OPC_KW_I : opclib/OPC Write  serverHost=localhost  serverID=OI.GATEWAY.3  itemIDs=Bucket Brigade.KW_I_LT401, Bucket Brigade.KW_I_LT401H, Bucket Brigade.KW_I_LT401L, Bucket Brigade.KW_I_TT402H, Bucket Brigade.KW_I_TT402M, Bucket Brigade.KW_I_TT402L, Bucket Brigade.KW_I_ST404, Bucket Brigade.KW_I_ET404, Bucket Brigade.KW_I_XV404Idle, Bucket Brigade.KW_I_XV404Running, Bucket Brigade.KW_I_XV404Alarm  writeMode=Synchronous  updateRate=1
  OPC_KZ_I : opclib/OPC Write  serverHost=localhost  serverID=OI.GATEWAY.3  itemIDs=Bucket Brigade.KZ_I_LT202, Bucket Brigade.KZ_I_LT202H, Bucket Brigade.KZ_I_LT202L, Bucket Brigade.KZ_I_FT201, Bucket Brigade.KZ_I_TT203H, Bucket Brigade.KZ_I_TT203M, Bucket Brigade.KZ_I_TT203L, Bucket Brigade.KZ_I_ST205, Bucket Brigade.KZ_I_ET205, Bucket Brigade.KZ_I_XV205Idle, Bucket Brigade.KZ_I_XV205Running, Bucket Brigade.KZ_I_XV205Alarm, Bucket Brigade.KZ_I_QT204  writeMode=Synchronous  updateRate=1
  OPC_MB_I : opclib/OPC Write  serverHost=localhost  serverID=OI.GATEWAY.3  itemIDs=Bucket Brigade.MB_I_FT105, Bucket Brigade.MB_I_LT102, Bucket Brigade.MB_I_LT102H, Bucket Brigade.MB_I_LT102L, Bucket Brigade.MB_I_ST103, Bucket Brigade.MB_I_ET103, Bucket Brigade.MB_I_FV103Idle, Bucket Brigade.MB_I_FV103Running, Bucket Brigade.MB_I_FV103Alarm, Bucket Brigade.MB_I_TT103, Bucket Brigade.MB_I_LT104H, Bucket Brigade.MB_I_LT104L, Bucket Brigade.MB_I_ST105, Bucket Brigade.MB_I_ET105, Bucket Brigade.MB_I_FV105Idle, Bucket Brigade.MB_I_FV105Running, Bucket Brigade.MB_I_FV105Alarm, Bucket Brigade.MB_I_TT105  writeMode=Synchronous  updateRate=1
  OPC_S_I : opclib/OPC Write  serverHost=localhost  serverID=Matrikon.OPC.Simulation.1  itemIDs=Bucket Brigade.S_I_TT601, Bucket Brigade.S_I_TT602, Bucket Brigade.S_I_TT603, Bucket Brigade.S_I_TT604  writeMode=Synchronous  updateRate=1
  wires:
  [FT105] -> Mux/1
  [LT102] -> Mux/2
  [LT102H] -> Mux/3
  [LT102L] -> Mux/4
  [ST103] -> Mux/5
  [ET103] -> Mux/6
  [FV103Idle] -> Mux/7
  [FV103Running] -> Mux/8
  [FV103Alarm] -> Mux/9
  [TT103] -> Mux/10
  [LT104H] -> Mux/11
  [LT104L] -> Mux/12
  [ST105] -> Mux/13
  [ET105] -> Mux/14
  [FV105dle] -> Mux/15
  [FV105Running] -> Mux/16
  [FV105Alarm] -> Mux/17
  [TT105] -> Mux/18
  Mux/1 -> OPC_MB_I/1
  [LT202] -> Mux1/1
  [LT202H] -> Mux1/2
  [LT202L] -> Mux1/3
  [FT201] -> Mux1/4
  [TT203H] -> Mux1/5
  [TT203M] -> Mux1/6
  [TT203L] -> Mux1/7
  [ST205] -> Mux1/8
  [ET205] -> Mux1/9
  [XV205Idle] -> Mux1/10
  [XV205Running] -> Mux1/11
  [XV205Alarm] -> Mux1/12
  [QT204] -> Mux1/13
  Mux1/1 -> OPC_KZ_I/1
  [LT308] -> Mux2/1
  [LT308H] -> Mux2/2
  [LT308L] -> Mux2/3
  [ST307] -> Mux2/4
  [ET307] -> Mux2/5
  [XV307Idle] -> Mux2/6
  [XV307Running] -> Mux2/7
  [XV307Alarm] -> Mux2/8
  [QT310] -> Mux2/9
  [LT309] -> Mux2/10
  [LT309H] -> Mux2/11
  [LT309L] -> Mux2/12
  [QT311] -> Mux2/13
  [QT312] -> Mux2/14
  [ST302] -> Mux2/15
  [ET302] -> Mux2/16
  [XV302Idle] -> Mux2/17
  [XV302Running] -> Mux2/18
  [XV302Alarm] -> Mux2/19
  [ST304] -> Mux2/20
  [ET304] -> Mux2/21
  [XV304Idle] -> Mux2/22
  [XV304Running] -> Mux2/23
  [XV304Alarm] -> Mux2/24
  Mux2/1 -> OPC_KF_I/1
  [LT401] -> Mux3/1
  [LT401H] -> Mux3/2
  [LT401L] -> Mux3/3
  [TT402H] -> Mux3/4
  [TT402M] -> Mux3/5
  [TT402L] -> Mux3/6
  [ST404] -> Mux3/7
  [ET404] -> Mux3/8
  [XV404Idle] -> Mux3/9
  [XV404Running] -> Mux3/10
  [XV404Alarm] -> Mux3/11
  Mux3/1 -> OPC_KW_I/1
  [LT502H] -> Mux4/1
  [LT502L] -> Mux4/2
  [PT503] -> Mux4/3
  [WT505] -> Mux4/4
  [XT504] -> Mux4/5
  [XT504C] -> Mux4/6
  [XT506H] -> Mux4/7
  [XT506L] -> Mux4/8
  Mux4/1 -> OPC_DCh_I/1
  [TT601] -> Mux5/1
  [TT602] -> Mux5/2
  [TT603] -> Mux5/3
  [TT604] -> Mux5/4
  Mux5/1 -> OPC_S_I/1
  [LT701] -> Mux6/1
  [LT701H] -> Mux6/2
  [LT701L] -> Mux6/3
  [TT702H] -> Mux6/4
  [TT702M] -> Mux6/5
  [TT702L] -> Mux6/6
  [ST704] -> Mux6/7
  [ET704] -> Mux6/8
  [XV704Idle] -> Mux6/9
  [XV704Running] -> Mux6/10
  [XV704Alarm] -> Mux6/11
  [ST705] -> Mux6/12
  [ET705] -> Mux6/13
  [XV705Idle] -> Mux6/14
  [XV705Running] -> Mux6/15
  [XV705Alarm] -> Mux6/16
  [Odplyw] -> Mux6/17
  Mux6/1 -> OPC_KFe_I/1
  [LT802H] -> Mux7/1
  [LT802L] -> Mux7/2
  [PT803] -> Mux7/3
  [WT805] -> Mux7/4
  [XT804] -> Mux7/5
  [XT804C] -> Mux7/6
  [XT806H] -> Mux7/7
  [XT806L] -> Mux7/8
  Mux7/1 -> OPC_DD_I/1

== system BrowarModel/System dozowania chmielu ==
  note: System dozowania chmielu
  LT502H : Subsystem
  LT502L : Subsystem
  LV501 : Subsystem
  PT503 : Subsystem  mask{SrcZakres=350, Zakres=350, Kompensacja=0, ZakloceniaPom=on}
      mask prompts: SrcZakres "Zakres zmiennej w modelu"; Zakres "Zakres pomiarowy przetwornika pomiarowego"; Kompensacja "Kompensacja przetwornika pomiarowego"; ZakloceniaPom "Zaklocenia pomiarowe"
  PV503 : Subsystem
  System dozowania chmielu : Subsystem
  WT505 : Subsystem  mask{SrcZakres=100, Zakres=100, Kompensacja=0, ZakloceniaPom=on}
      mask prompts: SrcZakres "Zakres zmiennej w modelu"; Zakres "Zakres pomiarowy przetwornika pomiarowego"; Kompensacja "Kompensacja przetwornika pomiarowego"; ZakloceniaPom "Zaklocenia pomiarowe"
  XT504 : Subsystem  mask{SrcZakres=0.1, Zakres=100, Kompensacja=0, ZakloceniaPom=on}
      mask prompts: SrcZakres "Zakres zmiennej w modelu"; Zakres "Zakres pomiarowy przetwornika pomiarowego"; Kompensacja "Kompensacja przetwornika pomiarowego"; ZakloceniaPom "Zaklocenia pomiarowe"
  XT504C : Subsystem
  XT506H : Subsystem
  XT506L : Subsystem
  XV504 : Subsystem
  XV506 : Subsystem
  Przeplyw chmielu : Outport
  tag scope: LT502H=global, LT502L=global, PT503=global, WT505=global, XT504=global, XT504C=global, XT506H=global, XT506L=global
  wires:
  LV501/1(Out) -> System dozowania chmielu/1(Doplyw zasobnika)
  PV503/1(Out) -> System dozowania chmielu/2(Zalaczenie pompy)
  XV504/1(Out) -> System dozowania chmielu/3(Sterowanie rusztem)
  System dozowania chmielu/1(Poziom wysoki zasobnika) -> LT502H/1(In)
  System dozowania chmielu/2(Poziom niski zasobnika) -> LT502L/1(In)
  System dozowania chmielu/3(Cisnienie pompy) -> PT503/1(In)
  System dozowania chmielu/4(Masa) -> WT505/1(In)
  XV506/1(Out) -> System dozowania chmielu/4(Oproznianie)
  System dozowania chmielu/5(Odplyw chmielu) -> Przeplyw chmielu/1
  LT502H/1(Out) -> [LT502H]
  LT502L/1(Out) -> [LT502L]
  PT503/1(Out) -> [PT503]
  WT505/1(Out) -> [WT505]
  XT504/1(Out) -> [XT504]
  System dozowania chmielu/6(Pozycja) -> XT504/1(In)
  XT504C/1(Out) -> [XT504C]
  System dozowania chmielu/7(PozycjaDisc) -> XT504C/1(In)
  XT506H/1(Out) -> [XT506H]
  System dozowania chmielu/8(Waga poz gora) -> XT506H/1(In)
  System dozowania chmielu/9(Waga poz dol) -> XT506L/1(In)
  XT506L/1(Out) -> [XT506L]

== system BrowarModel/System dozowania drozdzy ==
  note: System dozowania drozdzy
  LT802H : Subsystem
  LT802L : Subsystem
  LV801 : Subsystem
  PT803 : Subsystem  mask{SrcZakres=350, Zakres=350, Kompensacja=0, ZakloceniaPom=on}
      mask prompts: SrcZakres "Zakres zmiennej w modelu"; Zakres "Zakres pomiarowy przetwornika pomiarowego"; Kompensacja "Kompensacja przetwornika pomiarowego"; ZakloceniaPom "Zaklocenia pomiarowe"
  PV803 : Subsystem
  System dozowania drozdzy : Subsystem
  WT805 : Subsystem  mask{SrcZakres=100, Zakres=100, Kompensacja=0, ZakloceniaPom=on}
      mask prompts: SrcZakres "Zakres zmiennej w modelu"; Zakres "Zakres pomiarowy przetwornika pomiarowego"; Kompensacja "Kompensacja przetwornika pomiarowego"; ZakloceniaPom "Zaklocenia pomiarowe"
  XT804 : Subsystem  mask{SrcZakres=0.1, Zakres=100, Kompensacja=0, ZakloceniaPom=on}
      mask prompts: SrcZakres "Zakres zmiennej w modelu"; Zakres "Zakres pomiarowy przetwornika pomiarowego"; Kompensacja "Kompensacja przetwornika pomiarowego"; ZakloceniaPom "Zaklocenia pomiarowe"
  XT804C : Subsystem
  XT806H : Subsystem
  XT806L : Subsystem
  XV804 : Subsystem
  XV806 : Subsystem
  Przeplyw drozdzy : Outport
  tag scope: LT802H=global, LT802L=global, PT803=global, WT805=global, XT804=global, XT804C=global, XT806H=global, XT806L=global
  wires:
  LV801/1(Out) -> System dozowania drozdzy/1(Doplyw zasobnika)
  PV803/1(Out) -> System dozowania drozdzy/2(Zalaczenie pompy)
  XV804/1(Out) -> System dozowania drozdzy/3(Sterowanie rusztem)
  System dozowania drozdzy/1(Poziom wysoki zasobnika) -> LT802H/1(In)
  XV806/1(Out) -> System dozowania drozdzy/4(Oproznianie)
  System dozowania drozdzy/5(Odplyw drozdzy) -> Przeplyw drozdzy/1
  LT802H/1(Out) -> [LT802H]
  LT802L/1(Out) -> [LT802L]
  PT803/1(Out) -> [PT803]
  WT805/1(Out) -> [WT805]
  XT804/1(Out) -> [XT804]
  XT804C/1(Out) -> [XT804C]
  XT806H/1(Out) -> [XT806H]
  XT806L/1(Out) -> [XT806L]
  System dozowania drozdzy/2(Poziom niski zasobnika) -> LT802L/1(In)
  System dozowania drozdzy/3(Cisnienie pompy) -> PT803/1(In)
  System dozowania drozdzy/4(Masa) -> WT805/1(In)
  System dozowania drozdzy/6(Pozycja) -> XT804/1(In)
  System dozowania drozdzy/7(PozycjaDisc) -> XT804C/1(In)
  System dozowania drozdzy/8(Waga poz gora) -> XT806H/1(In)
  System dozowania drozdzy/9(Waga poz dol) -> XT806L/1(In)

== system BrowarModel/Kadz fermentacyjna/ET704 ==
  note: Przetwornik pomiarowy
  In : Inport
  F_gain : Gain  Gain=0
  F_offset : Constant  Value=0
  GUIMon : Gain
  Kompensacja : Constant  Value=Kompensacja
  Product : Product  RndMeth=Zero
  Saturation : Saturate  UpperLimit=100  LowerLimit=0
  Skalowanie (0-100%) : Gain  Gain=100/SrcZakres
  Sum{,1..3} (4 alike) : Sum  Inputs=|++
  Transfer Fcn : TransferFcn  Denominator=[0.3 1]
  Zaklocenia pomiarowe : Subsystem
  Zakres : Constant  Value=Zakres/100
  Out : Outport
  wires:
  Transfer Fcn/1 -> Saturation/1
  F_offset/1 -> Sum3/2
  F_gain/1 -> Sum2/2
  Product/1 -> Sum/1
  Zakres/1 -> Product/2
  Kompensacja/1 -> Sum/2
  Sum/1 -> GUIMon/1
  Skalowanie (0-100%)/1 -> Sum1/1
  Zaklocenia pomiarowe/1(Out) -> Sum1/2
  Sum1/1 -> F_gain/1, Sum2/1
  Sum3/1 -> Transfer Fcn/1
  Sum2/1 -> Sum3/1
  In/1 -> Skalowanie (0-100%)/1
  GUIMon/1 -> Out/1
  Saturation/1 -> Product/1
